simulink model "cic_decimator"  (Simulink 6.6)
settings: Solver=VariableStepDiscrete  SolverMode=SingleTasking  StartTime=0.0  StopTime=1024/10e6  RelTol=1e-3
StopFcn:
  | doFFTplot((10e6)/16,[CIC1],['CIC1'],16)
libraries: xbsIndex_r4 x26, dspsrcs4 x1
settings Model: Creator=lcrockett  LastModifiedBy=lcrockett
settings DataIOCC: SignalLoggingName=sigsOut
settings OptimizationCC: InlineParams=on  InlineInvariantSignals=on
settings DebuggingCC: SignalResolutionControl=TryResolveAllWithWarning  SolverPrmCheckMsg=none  MultiTaskDSMMsg=warning  MultiTaskCondExecSysMsg=none  StrictBusMsg=None
settings HardwareCC: TargetUnknown=on
settings RTWCC: IncludeERTFirstTime=on
settings GRTTargetCC: ModelReferenceCompliant=off  MatFileLogging=off

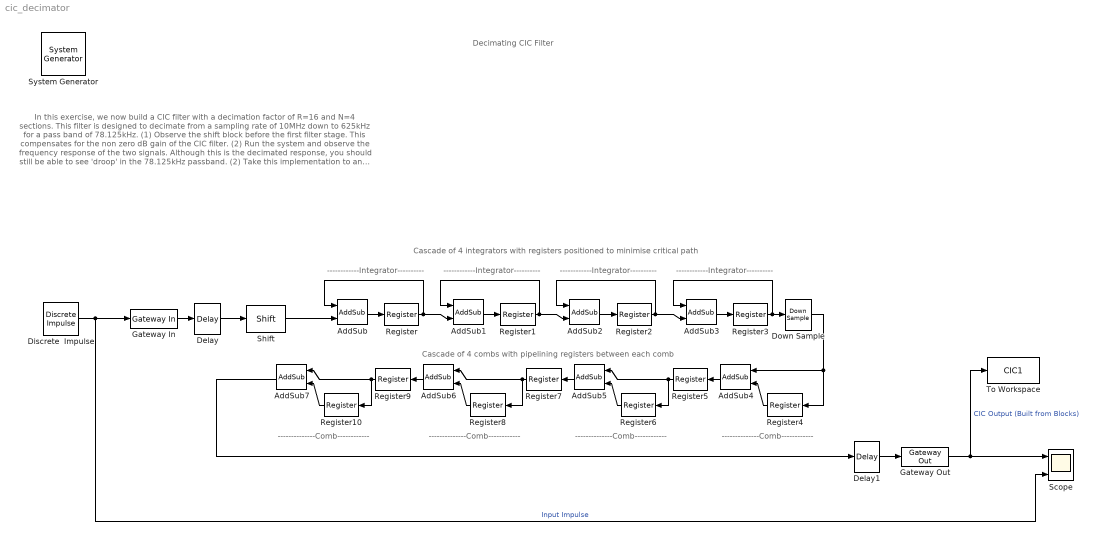
== system cic_decimator ==
  note: ------------Integrator----------
  note: In this exercise, we now build a CIC filter with a decimation factor of R=16 and N=4 sections.
      | This filter is designed to decimate from a sampling rate of 10MHz down to 625kHz for a pass band of 78.125kHz.
      |
      | (1) Observe the shift block before the first filter stage.  This compensates for the non zero dB gain of the CIC filter.
      |
      | (2) Run the system and observe the frequency response of the two signals.  Although this is the decimated response, you should
      | still be able to see 'droop' in the 78.125kHz passband.
      |
      | (2) Take this implementation to an FPGA design using the XC2VP30 from the Virtex II Pro family.
      | Note that for obvious reasons there are no block multipliers to be used in the implementation.
  note: Decimating CIC Filter
  note: ------------Integrator----------
  note: ------------Integrator----------
  note: ------------Integrator----------
  note: --------------Comb------------
  note: --------------Comb------------
  note: --------------Comb------------
  note: --------------Comb------------
  note: Cascade of 4 integrators with registers positioned to minimise critical path
  note: Cascade of 4 combs with pipelining registers between each comb
  " System Generator" : xbsIndex_r4/ System Generator  Tag=genX  SystemSampleTime=-1  xilinxfamily=virtex2p  part=xc2vp30  speed=-7  package=ff896  synthesis_tool=XST  clock_wrapper=Clock Enables  directory=./netlist  testbench=off  simulink_period=1/10e6  sysclk_period=100  dcm_input_clock_period=100  incr_netlist=off  trim_vbits=Everywhere in SubSystem  dbl_ovrd=According to Block Masks  core_generation=According to Block Masks  run_coregen=off  deprecated_control=off  eval_field=0  block_type=sysgen
      settings: block_version=8.2
  AddSub{,1..3} (4 alike) : xbsIndex_r4/AddSub  mode=Addition  use_carryin=off  use_carryout=off  en=off  latency=0  precision=User Defined  arith_type="Signed  (2's comp)"  n_bits=18  bin_pt=16  quantization=Truncate  overflow=Wrap  dbl_ovrd=off  use_behavioral_HDL=on  pipelined=off  use_rpm=on  block_type=addsub
      settings: xl_area=[0, 0, 0, 0, 0, 0, 0]  block_version=VER_STRING_GOES_HERE
  AddSub{4..7} (4 alike) : xbsIndex_r4/AddSub  Orientation=left  mode=Subtraction  use_carryin=off  use_carryout=off  en=off  latency=0  precision=User Defined  arith_type="Signed  (2's comp)"  n_bits=18  bin_pt=16  quantization=Truncate  overflow=Wrap  dbl_ovrd=off  use_behavioral_HDL=on  pipelined=off  use_rpm=on  block_type=addsub
      settings: xl_area=[0, 0, 0, 0, 0, 0, 0]  block_version=VER_STRING_GOES_HERE
  Delay : xbsIndex_r4/Delay  en=off  latency=1  dbl_ovrd=off  reg_retiming=off  block_type=delay
      settings: block_version=10.1.2
  Delay1 : xbsIndex_r4/Delay  en=off  latency=1  dbl_ovrd=off  reg_retiming=off  block_type=delay
      settings: block_version=10.1.2
  Discrete  Impulse : dspsrcs4/Discrete  Impulse  Delay=0  SampleTime=1/10e6  FrameSample=1  dataType=double  isSigned=on  wordLen=16  udDataType=sfix(16)  fracBitsMode=Best precision  numFracBits=14
  Down Sample : xbsIndex_r4/Down Sample  sample_ratio=16  sample_phase="Last Value of Frame  (most efficient)"  en=off  latency=1  dbl_ovrd=off  block_type=dsamp
      settings: xl_area=[0, 0, 0, 0, 0, 0, 0]  block_version=VER_STRING_GOES_HERE
  Gateway In : xbsIndex_r4/Gateway In  arith_type="Signed  (2's comp)"  n_bits=18  bin_pt=16  quantization=Truncate  overflow=Wrap  period=1/10e6  dbl_ovrd=off  timing_constraint=None  locs_specified=off  LOCs={}  block_type=gatewayin
      settings: infoedit="Gateway in block.  Converts inputs of type Simulink integer, double and fixed point to  Xilinx fixed point type.<P><P>Hardware notes:  In hardware these blocks become top level input ports."  xl_area=[0, 0, 0, 0, 0, 0, 0]  block_version=VER_STRING_GOES_HERE
  Gateway Out : xbsIndex_r4/Gateway Out  hdl_port=on  timing_constraint=None  locs_specified=off  LOCs={}  block_type=gatewayout
      settings: infoedit="Gateway out block.  Converts Xilinx fixed point inputs into ouputs of type Simulink integer, double, or fixed point.<P><P>Hardware notes:  In hardware these blocks become top level output ports or are discarded, depending on how they are configured."  xl_area=[0, 0, 0, 0, 0, 0, 0]  block_version=VER_STRING_GOES_HERE
  Register{,1..3} (4 alike) : xbsIndex_r4/Register  init=0  rst=off  en=off  dbl_ovrd=off  block_type=register
      settings: xl_area=[0, 0, 0, 0, 0, 0, 0]  block_version=VER_STRING_GOES_HERE
  Register{4..10} (7 alike) : xbsIndex_r4/Register  Orientation=left  init=0  rst=off  en=off  dbl_ovrd=off  block_type=register
      settings: xl_area=[0, 0, 0, 0, 0, 0, 0]  block_version=VER_STRING_GOES_HERE
  Scope : Scope  NumInputPorts=2
      settings: TimeRange=0.00012  YMin=0~0  YMax=3000~3000
  Shift : xbsIndex_r4/Shift  shift_dir=Right  shift_bits=16  en=off  latency=0  precision=Full  arith_type="Signed  (2's comp)"  n_bits=8  bin_pt=2  quantization=Truncate  overflow=Wrap  dbl_ovrd=off  block_type=shift
      settings: xl_area=[0, 0, 0, 0, 0, 0, 0]  block_version=VER_STRING_GOES_HERE
  To Workspace : ToWorkspace  VariableName=CIC1  SampleTime=-1  SaveFormat=Array
  wires:
  Gateway In/1 -> Delay/1
  Gateway Out/1 -> Scope/1, To Workspace/1  "CIC Output (Built from Blocks)"
  AddSub/1 -> Register/1
  Register/1 -> AddSub/1, AddSub1/2
  Discrete  Impulse/1 -> Gateway In/1, Scope/2  "Input Impulse"
  AddSub1/1 -> Register1/1
  Register1/1 -> AddSub1/1, AddSub2/2
  AddSub2/1 -> Register2/1
  Register2/1 -> AddSub2/1, AddSub3/2
  AddSub3/1 -> Register3/1
  Register3/1 -> AddSub3/1, Down Sample/1
  Down Sample/1 -> AddSub4/1, Register4/1
  Register4/1 -> AddSub4/2
  AddSub4/1 -> Register5/1
  Register5/1 -> AddSub5/1, Register6/1
  Register6/1 -> AddSub5/2
  AddSub5/1 -> Register7/1
  Register7/1 -> AddSub6/1, Register8/1
  Register8/1 -> AddSub6/2
  AddSub6/1 -> Register9/1
  Register9/1 -> AddSub7/1, Register10/1
  Register10/1 -> AddSub7/2
  AddSub7/1 -> Delay1/1
  Shift/1 -> AddSub/2
  Delay/1 -> Shift/1
  Delay1/1 -> Gateway Out/1
